simulink model "Sampling_wAliasing_AudioToolbox_b"  (R2016a)
settings: Solver=VariableStepAuto  StartTime=0.0  StopTime=inf  RelTol=1e-3
libraries: audiosources x1, dspsnks4 x1, dsparch4 x1, dspsigops x1
settings Model: Creator=Student  LastModifiedBy=Student

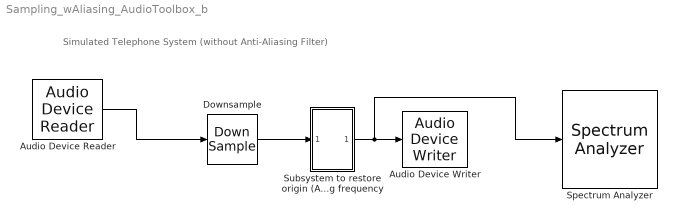
== system Sampling_wAliasing_AudioToolbox_b ==
  note: Simulated Telephone System (without Anti-Aliasing Filter)
  Audio Device Reader : audiosources/Audio Device Reader  Driver=DirectSound  Device=Default  SampleRate=48000  NumChannels=1  SamplesPerFrame=60  BitDepth=16-bit integer  NumBuffers=10  DefaultInputChannelMapping=on  InputChannelMapping=1:2  OutputNumOverrunSamples=off  OutputDataType=double  DriverIdx=1  DeviceWarnFlag=''
  Audio Device Writer : dspsnks4/Audio Device Writer  Driver=DirectSound  Device=Default  InheritSampleRate=on  SampleRate=44100  BitDepth=16-bit integer  BufferSize=4096  NumBuffers=10  DefaultOutputChannelMapping=on  OutputChannelMapping=1:2  OutputNumUnderrunSamples=off  DriverIdx=1  DeviceWarnFlag=''
  Downsample : DownSample  N=6
  Spectrum Analyzer : SpectrumAnalyzer
  Subsystem to restore origin (ADC) sampling frequency : Subsystem
  wires:
  Downsample/1 -> Subsystem to restore origin (ADC) sampling frequency/1(In1)
  Subsystem to restore origin (ADC) sampling frequency/1(Out1) -> Spectrum Analyzer/1, Audio Device Writer/1
  Audio Device Reader/1 -> Downsample/1

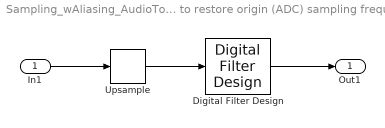
== system Sampling_wAliasing_AudioToolbox_b/Subsystem to restore origin (ADC) sampling frequency ==
  In1 : Inport
  Digital Filter Design : dsparch4/Digital Filter Design  mwdsp_browser_bugfix_var=off
  Upsample : dspsigops/Upsample  N=6  phase=0  InputProcessing=Columns as channels (frame based)  RateOptions=Enforce single-rate processing  ic=0  mode=Unused parameter value
  Out1 : Outport
  wires:
  In1/1 -> Upsample/1
  Upsample/1 -> Digital Filter Design/1
  Digital Filter Design/1 -> Out1/1
